simulink model "SoleusMuscleEnergyTest"  (R2019b)
settings: Solver=ode15s  StartTime=0.0  StopTime=11  MaxStep=0.01  RelTol=1e-4  AbsTol=1e-6
values from neighbouring files (symbols this model uses):
  FmaxSOL = 4000    [BodyMechParams.m]
  FT_SOL = 11    [BodyMechParams.m]
  loptSOL = 0.04    [BodyMechParams.m]
  lslackSOL = 0.26    [BodyMechParams.m]
  vmaxSOL = 6    [BodyMechParams.m]
libraries: NeuroMuscularLibrary x2, simulink x1
settings Model: Creator=Nathan  LastModifiedBy=Nathan
settings DataIOCC: SaveFinalState=on  SaveFormat=StructureWithTime  SaveOutput=off  SaveState=on  ReturnWorkspaceOutputs=off

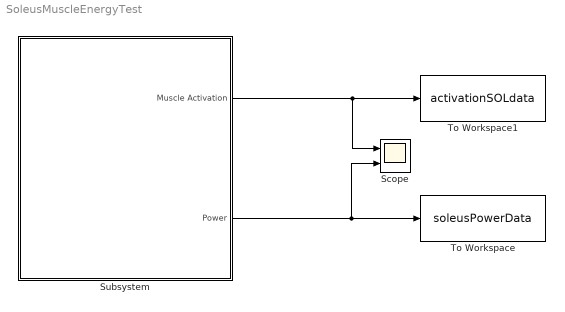
== system SoleusMuscleEnergyTest ==
  Scope : Scope  NumInputPorts=2
  Subsystem : Subsystem  mask{Fmax=FmaxSOL, lopt=loptSOL, vmax=vmaxSOL, lslack=lslackSOL, FT=FT_SOL, iso_short_length=Lengthening}
      mask prompts: Fmax "Max Isometric Force in N"; lopt "Optimal Length in m"; vmax "Max Contraction Velocity in m/s"; lslack "Slack Length [m]"; FT "Percent Fast Twitch"; iso_short_length "Type of muscle movement"
      mask TypeOptions iso_short_length: Lengthening | Isometric | Shortening
  To Workspace : ToWorkspace  VariableName=soleusPowerData  SampleTime=-1
  To Workspace1 : ToWorkspace  VariableName=activationSOLdata  SampleTime=-1
  wires:
  Subsystem/2(Power) -> Scope/2, To Workspace/1
  Subsystem/1(Muscle Activation) -> Scope/1, To Workspace1/1

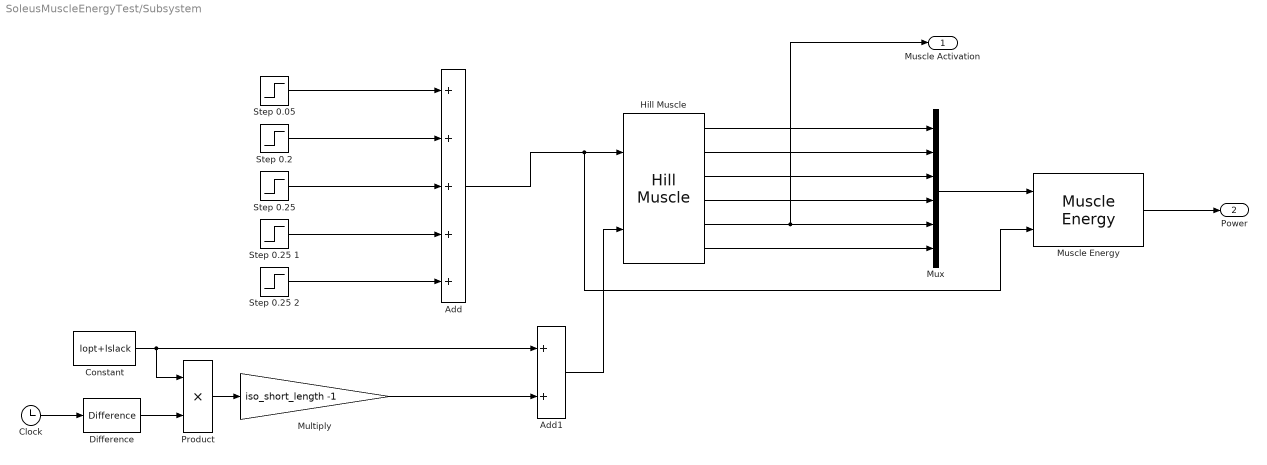
== system SoleusMuscleEnergyTest/Subsystem ==
  Add : Sum  Inputs=+++++
  Add1 : Sum
  Clock : Clock
  Constant : Constant  Value=lopt+lslack
  Difference : simulink/Discrete/Difference  ICPrevInput=0.0  OutMin=[]  OutMax=[]  OutDataType=fixdt(1, 16)  OutScaling=2^-10  DoSatur=off
  Hill Muscle : NeuroMuscularLibrary/Hill Muscle  Fmax=Fmax  lopt=lopt  vmax=vmax  lslack=lslack
  Multiply : Gain  Gain=iso_short_length -1
  Muscle Energy : NeuroMuscularLibrary/Muscle Energy  lopt=lopt  FT=FT  Fmax=Fmax
  Mux : Mux  Inputs=6
  Product : Product
  Step 0.05 : Step  After=0.05  SampleTime=0
  Step 0.2 : Step  Time=3  After=0.2  SampleTime=0
  Step 0.25 : Step  Time=5  After=0.25  SampleTime=0
  Step 0.25 1 : Step  Time=7  After=0.25  SampleTime=0
  Step 0.25 2 : Step  Time=9  After=0.25  SampleTime=0
  Muscle Activation : Outport
  Power : Outport  Port=2
  wires:
  Mux/1 -> Muscle Energy/1
  Add/1 -> Muscle Energy/2, Hill Muscle/1
  Hill Muscle/3 -> Mux/3
  Hill Muscle/4 -> Mux/4
  Hill Muscle/6 -> Mux/6
  Hill Muscle/2 -> Mux/2
  Step 0.25 1/1 -> Add/4
  Hill Muscle/1 -> Mux/1
  Hill Muscle/5 -> Muscle Activation/1, Mux/5
  Step 0.2/1 -> Add/2
  Step 0.25 2/1 -> Add/5
  Step 0.25/1 -> Add/3
  Step 0.05/1 -> Add/1
  Muscle Energy/1 -> Power/1
  Constant/1 -> Product/1, Add1/1
  Add1/1 -> Hill Muscle/2
  Clock/1 -> Difference/1
  Product/1 -> Multiply/1
  Difference/1 -> Product/2
  Multiply/1 -> Add1/2
